simulink model "get_phi"  (R2015b)
settings: Solver=ode45  StartTime=0.0  StopTime=10.0  RelTol=1e-3
libraries: cstblocks x2
settings Model: Creator=Christoph Zech  LastModifiedBy=danielhauer
settings DataIOCC: SaveFormat=Array
settings DebuggingCC: UnderspecifiedInitializationDetection=Classic  MergeDetectMultiDrivingBlocksExec=none  SolverPrmCheckMsg=warning  StateNameClashWarn=warning
settings HardwareCC: ProdBitPerPointer=32  ProdLargestAtomicFloat=None  ProdIntDivRoundTo=Undefined  ProdEndianess=Unspecified  ProdWordSize=32  ProdHWDeviceType=32-bit Generic
settings GRTTargetCC: GeneratePreprocessorConditionals=Disable all
settings ConfigComp: CovModelRefEnable=Off

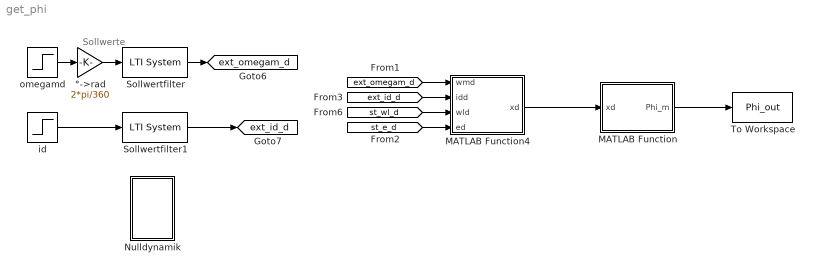
== system get_phi ==
  note: Sollwerte
  MATLAB Function : MATLAB Function  TreatAsAtomicUnit=on
  MATLAB Function4 : MATLAB Function  TreatAsAtomicUnit=on
  Nulldynamik : Subsystem
  Sollwertfilter : cstblocks/LTI System  sys=parReg.ssSF  IC=[]
  Sollwertfilter1 : cstblocks/LTI System  sys=parReg.ssSFi  IC=[]
  To Workspace : ToWorkspace  VariableName=Phi_out  SaveFormat=Timeseries  SampleTime=-1
  id : Step  Time=0.5  After=0.1  SampleTime=0
  omegamd : Step  Time=2  After=1000/60*360  SampleTime=0
  °->rad : Gain  Gain=2*pi/360
  tag scope: ext_id_d=global, ext_omegam_d=global
  wires:
  °->rad/1 -> Sollwertfilter/1
  Sollwertfilter/1 -> [ext_omegam_d]
  Sollwertfilter1/1 -> [ext_id_d]
  id/1 -> Sollwertfilter1/1
  omegamd/1 -> °->rad/1
  MATLAB Function/1(Phi_m) -> To Workspace/1
  MATLAB Function4/1(xd) -> MATLAB Function/1(xd)
  [ext_omegam_d] -> MATLAB Function4/1(wmd)
  [st_wl_d] -> MATLAB Function4/3(wld)
  [st_e_d] -> MATLAB Function4/4(ed)
  [ext_id_d] -> MATLAB Function4/2(idd)

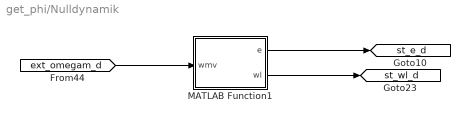
== system get_phi/Nulldynamik ==
  MATLAB Function1 : MATLAB Function  TreatAsAtomicUnit=on
  tag scope: st_e_d=global, st_wl_d=global
  wires:
  MATLAB Function1/1(e) -> [st_e_d]
  MATLAB Function1/2(wl) -> [st_wl_d]
  [ext_omegam_d] -> MATLAB Function1/1(wmv)

== matlab function get_phi/MATLAB Function ==
  settings: updateMethod=DISCRETE  sampleTime=parSys.TsID
  data: xd input; Phi_m output
function Phi_m = fcn(xd)
%#codegen
%Parameter
I_l  = 4e-5;     %Trägheitsmoment Last
cr1 = 10;       %lineare Steifigkeit Riemen
cr3 = 1e6;      %kubische Steifigkeit Riemen (1e6)
dl  = 0.001;    %visk. Dämpfung Last
rl  = 0.05;     %Radius Riemenscheibe Last
I_m  = 0.5e-5;   %Trägheitsmoment Motor
dm  = 0.01;     %viskose Dämpfung Motor
rm  = 0.025;    %Radius Riemenscheibe Motor
Rm  = 1.388;    %Widerstand PSM
Lm  = 1.475e-3; %Induktivität PSM
p   = 2.0;      %Polpaarzahl PSM
Phi = 2.715e-2; %Fluss Permanentmagnet PSM

Ta = 0.1e-3;

wm_d = xd(1);
iq_d = xd(2);
id_d = xd(3);
e_d = xd(4);
wl_d = xd(5);

Phi_m = [1 - Ta * dm / I_m 0.3e1 / 0.2e1 * Ta * Phi * p / I_m 0 (Ta * (12 * cr3 * e_d ^ 2 * rm + 4 * cr1 * rm) / I_m) / 0.2e1 0 0 0; (Ta * (3 * Lm * id_d * p - 2 * Phi * p) / Lm) / 0.3e1 0.1e1 - 0.2e1 / 0.3e1 * Ta * Rm / Lm Ta * p * wm_d 0 0 0 0; -Ta * iq_d * p -Ta * p * wm_d 0.1e1 - 0.2e1 / 0.3e1 * Ta * Rm / Lm 0 0 0 0; -Ta * rm 0 0 1 Ta * rl 0 0; 0 0 0 -Ta * (6 * cr3 * e_d ^ 2 * rl + 2 * cr1 * rl) / I_l 1 - Ta * dl / I_l 0 0; Ta 0 0 0 0 1 0; 0 0 Ta 0 0 0 1;];
end

== matlab function get_phi/Nulldynamik/MATLAB Function1 ==
  settings: updateMethod=DISCRETE  sampleTime=parSys.TsID
  data: wmv input; e output; wl output; parSys parameter
function [e, wl] = Null_disc(wmv, parSys)
%#codegen
persistent k
persistent x1
persistent x2
persistent wm_old

wm = wmv(1);


if (isempty(k))
    k = 0;
end
if (isempty(x1))
    x1 = parSys.eta_1_0;
end
if (isempty(x2))
    x2 = parSys.eta_2_0;
end
if (isempty(wm_old))
    wm_old = 0;
end

cr1 = parSys.cr1;
cr3 = parSys.cr3;
Il = parSys.Il;
rl = parSys.rl;
rm = parSys.rm;
dl = parSys.dl;

k = k + parSys.TsID;

f1 = rl*x2-rm*wm_old;
f2 = 1/Il*(-2*(cr1*x1+cr3*x1^3)*rl - dl*x2);

xp1 = x1 + parSys.TsID*f1;
xp2 = x2 + parSys.TsID*f2;

x1 = x1 + parSys.TsID/2*(f1 + (rl*xp2 - rm*wm));
x2  = x2 + parSys.TsID/2*(f2 + 1/Il*(-2*(cr1*xp1 + cr3*xp1^3)*rl - dl*xp2));

e = x1;
wl = x2;

wm_old = wm;
end

== matlab function get_phi/MATLAB Function4 ==
  data: wmd input; idd input; xd output; wld input; ed input; parSys parameter
function xd  = fcn(wmd, idd, wld, ed, parSys)
%#codegen
wm = wmd(1);
wmp = wmd(2);
wmpp = wmd(3);
id = idd(1);
idp = idd(2);
wl = wld;
e = ed;

%parameter;
%Zuweisungen
Lm = parSys.Lm;
Rm = parSys.Rm;
cr1 = parSys.cr1;
cr3 = parSys.cr3;
rm = parSys.rm;
dm = parSys.dm;
rl = parSys.rl;
dl = parSys.dl;
I_l = parSys.Il;
I_m = parSys.Im;
p = parSys.p;
Phi = parSys.Phi;

iq = 0.2e1 / 0.3e1 * (-2 * cr3 * e ^ 3 * rm - 2 * cr1 * e * rm + wmp * I_m + dm * wm) / Phi / p;

xd = [wm iq id e wl];


end
